simulink model "model"  (R2015a)
settings: Solver=ode45  StartTime=0.0  StopTime=50  RelTol=1e-3
values from neighbouring files (symbols this model uses):
  A = [-R/L,0,0; 0,0,1; 1/L, -Kh/M, -Ch/M]    [script.m]
  B = [1;0;0]    [script.m]
  C = [0,-10^5/M,0]    [script.m]
  Ch = 9    [script.m]
  D = 0    [script.m]
  Kh = 625    [script.m]
  Kx = place(A,B,[-60, -50,-40])    [script.m]
  L = 0.0220    (= 0.022)    [script.m]
  Lx = place(A',C',[-600,-500,-400])'    [script.m]
  M = 1.35    [script.m]
  R = 1.3    [script.m]
settings Model: Creator=jinkale  LastModifiedBy=jinkale

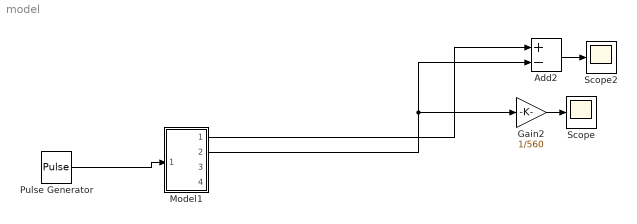
== system model ==
  Add2 : Sum  Inputs=+-
  Gain2 : Gain  Gain=1/560
  Model1 : Subsystem
  Pulse Generator : DiscretePulseGenerator  PulseType=Time based  Period=3  PulseWidth=50  PhaseDelay=10
  Scope : Scope
  Scope2 : Scope
      settings: TimeRange=27.63918388123077  YMin=-600  YMax=100  SaveName=ScopeData2
  wires:
  Add2/1 -> Scope2/1
  Gain2/1 -> Scope/1
  Model1/2(Out2) -> Add2/2, Gain2/1
  Model1/1(Out1) -> Add2/1
  Pulse Generator/1 -> Model1/1(In1)

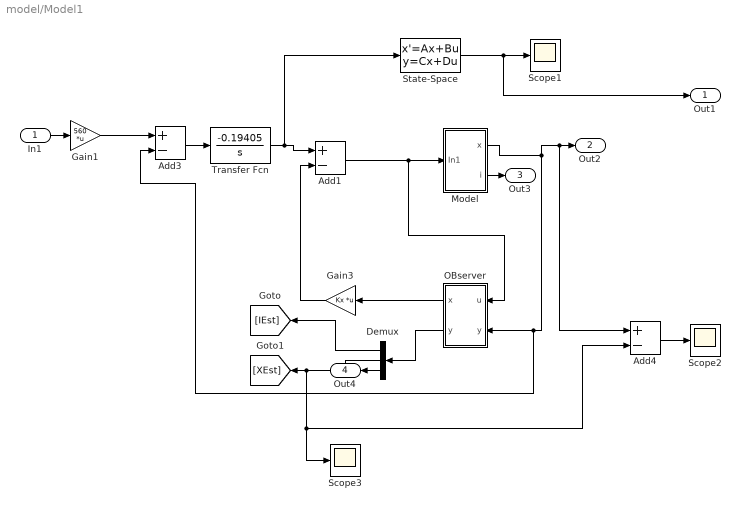
== system model/Model1 ==
  In1 : Inport
  Add1 : Sum  Inputs=+-
  Add3 : Sum  Inputs=+-
  Add4 : Sum  Inputs=+-
  Demux : Demux  Outputs=3
  Gain1 : Gain  Gain=560  Multiplication=Matrix(K*u) (u vector)
  Gain3 : Gain  Gain=Kx  Multiplication=Matrix(K*u)
  Model : Subsystem
  OBserver : Subsystem
  Scope1 : Scope
  Scope2 : Scope
      settings: SaveName=ScopeData5
  Scope3 : Scope
      settings: SaveName=ScopeData4
  State-Space : StateSpace  A=A-B*Kx  B=B  C=C  D=D  X0=0
  Transfer Fcn : TransferFcn  Numerator=[-0.19405]  Denominator=[1 0]
  Out1 : Outport
  Out2 : Outport  Port=2
  Out3 : Outport  Port=3
  Out4 : Outport  Port=4
  wires:
  Transfer Fcn/1 -> State-Space/1, Add1/1
  Gain1/1 -> Add3/1
  Add3/1 -> Transfer Fcn/1
  Demux/3 -> Out4/1
  OBserver/2("y ") -> Demux/1
  Model/1(x) -> Add4/1, Out2/1, Add3/2, OBserver/2(y)
  Add1/1 -> Model/1(In1), OBserver/1(u)
  Demux/2 -> Add4/2, Scope3/1, [XEst]
  Gain3/1 -> Add1/2
  Model/2(i) -> Out3/1
  State-Space/1 -> Out1/1, Scope1/1
  Demux/1 -> [IEst]
  In1/1 -> Gain1/1
  OBserver/1("x ") -> Gain3/1
  Add4/1 -> Scope2/1

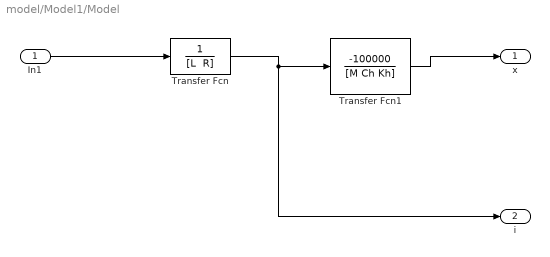
== system model/Model1/Model ==
  In1 : Inport
  Transfer Fcn : TransferFcn  Denominator="[L  R]"
  Transfer Fcn1 : TransferFcn  Numerator=[-100000]  Denominator=[M Ch Kh]
  x : Outport
  i : Outport  Port=2
  wires:
  Transfer Fcn/1 -> i/1, Transfer Fcn1/1
  In1/1 -> Transfer Fcn/1
  Transfer Fcn1/1 -> x/1

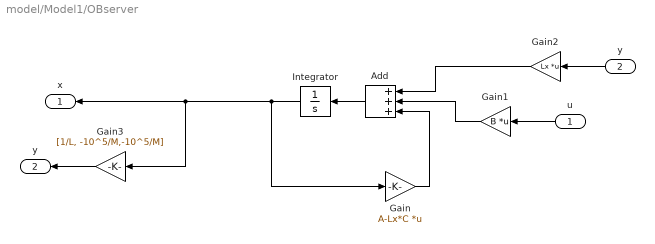
== system model/Model1/OBserver ==
  u : Inport
  y : Inport  Port=2
  Add : Sum  Inputs=+++
  Gain : Gain  Gain=A-Lx*C  Multiplication=Matrix(K*u)
  Gain1 : Gain  Gain=B  Multiplication=Matrix(K*u)
  Gain2 : Gain  Gain=Lx  Multiplication=Matrix(K*u)
  Gain3 : Gain  Gain=[1/L, -10^5/M,-10^5/M]
  Integrator : Integrator
  "x " : Outport
  "y " : Outport  Port=2
  wires:
  Add/1 -> Integrator/1
  Integrator/1 -> Gain/1, Gain3/1, "x "/1
  Gain/1 -> Add/3
  Gain1/1 -> Add/2
  Gain2/1 -> Add/1
  y/1 -> Gain2/1
  u/1 -> Gain1/1
  Gain3/1 -> "y "/1
